simulink model "Quadcopter_Hinfinity"  (R2016b)
settings: Solver=ode45  StartTime=0.0  StopTime=36  RelTol=1e-3  EnableMultiTasking=on
undefined symbols (not defined in the file): A, B, C, D, K1
libraries: simulink x1
settings Model: Creator=Toshiba  LastModifiedBy=AAstudillo
settings DataIOCC: LimitDataPoints=on  SaveFormat=Array  SignalLoggingSaveFormat=ModelDataLogs
settings OptimizationCC: LifeSpan=inf
settings DebuggingCC: SolverPrmCheckMsg=warning  MultiTaskDSMMsg=warning  MultiTaskCondExecSysMsg=none  SFUnexpectedBacktrackingDiag=warning  SFNoUnconditionalDefaultTransitionDiag=warning  SFExecutionAtInitializationDiag=none
settings HardwareCC: ProdBitPerPointer=32  ProdBitPerSizeT=32  ProdBitPerPtrDiffT=32  ProdLargestAtomicFloat=None  ProdIntDivRoundTo=Undefined  ProdEndianess=Unspecified  ProdWordSize=32  ProdHWDeviceType=32-bit Generic
settings ModelReferenceCC: PropagateSignalLabelsOutOfModel=off
settings GRTTargetCC: TargetLangStandard=C89/C90 (ANSI)  GeneratePreprocessorConditionals=Disable all
settings ConfigComp: CovMetricSettings=dw  CovHtmlReporting=on  CovSaveCumulativeToWorkspaceVar=on  CovSaveSingleToWorkspaceVar=on  CovExternalEMLEnable=off

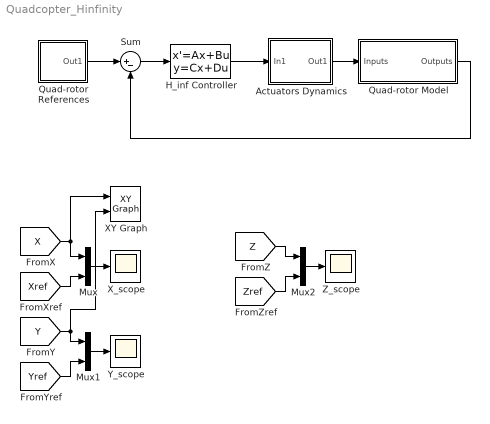
== system Quadcopter_Hinfinity ==
  Actuators Dynamics : Subsystem
  H_inf Controller : StateSpace  A=K1.a  B=K1.b  C=K1.c  D=K1.d  X0=zeros(size(K1.a,1),1)
  Mux : Mux  Inputs=2
  Mux1 : Mux  Inputs=2
  Mux2 : Mux  Inputs=2
  Quad-rotor Model : Subsystem
  Quad-rotor References : Subsystem
  Sum : Sum  Inputs=|+-
  XY Graph : simulink/Sinks/XY Graph  xmin=-1  xmax=1  ymin=-1  ymax=1  st=-1
  X_scope : Scope
  Y_scope : Scope
  Z_scope : Scope
  wires:
  Sum/1 -> H_inf Controller/1
  Quad-rotor References/1(Out1) -> Sum/1
  Quad-rotor Model/1(Outputs) -> Sum/2
  Mux/1 -> X_scope/1
  Mux1/1 -> Y_scope/1
  Mux2/1 -> Z_scope/1
  [X] -> Mux/1, XY Graph/1
  [Xref] -> Mux/2
  [Y] -> Mux1/1, XY Graph/2
  [Yref] -> Mux1/2
  [Z] -> Mux2/1
  [Zref] -> Mux2/2
  H_inf Controller/1 -> Actuators Dynamics/1(In1)
  Actuators Dynamics/1(Out1) -> Quad-rotor Model/1(Inputs)

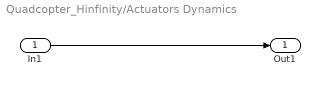
== system Quadcopter_Hinfinity/Actuators Dynamics ==
  In1 : Inport
  Out1 : Outport
  wires:
  In1/1 -> Out1/1

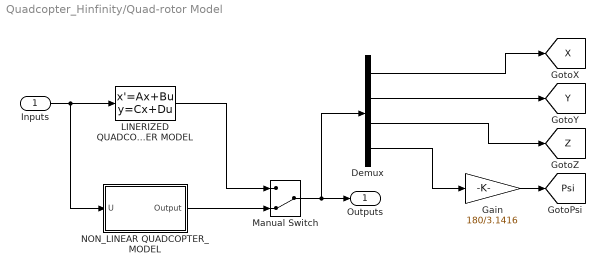
== system Quadcopter_Hinfinity/Quad-rotor Model ==
  Inputs : Inport
  Demux : Demux
  Gain : Gain  Gain=180/3.1416
  LINERIZED QUADCOPTER MODEL : StateSpace  A=A  B=B  C=C  D=D  X0=[0 0 1 0 1.5 0 45*pi/180 0 0 0 0 0]'
  Manual Switch : ManualSwitch  CurrentSetting=0
  NON_LINEAR QUADCOPTER_MODEL : Subsystem
  Outputs : Outport
  tag scope: Psi=global, X=global, Y=global, Z=global
  wires:
  Inputs/1 -> NON_LINEAR QUADCOPTER_MODEL/1(U), LINERIZED QUADCOPTER MODEL/1
  LINERIZED QUADCOPTER MODEL/1 -> Manual Switch/1
  Demux/3 -> [Z]
  Manual Switch/1 -> Outputs/1, Demux/1
  Demux/1 -> [X]
  Demux/2 -> [Y]
  NON_LINEAR QUADCOPTER_MODEL/1("Output ") -> Manual Switch/2
  Gain/1 -> [Psi]
  Demux/4 -> Gain/1

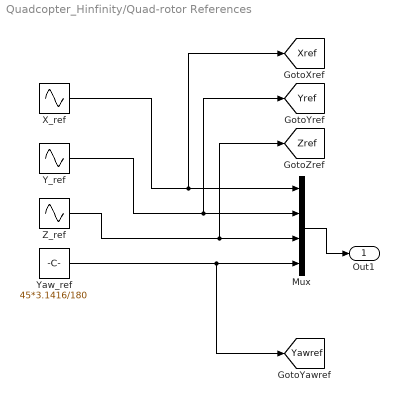
== system Quadcopter_Hinfinity/Quad-rotor References ==
  Mux : Mux
  X_ref : Sin  Frequency=3.141592654*0.1  SampleTime=0
  Y_ref : Sin  Frequency=3.141592654*0.1  Phase=3.141592654/2  SampleTime=0
  Yaw_ref : Constant  Value=45*3.1416/180
  Z_ref : Sin  Bias=1  Frequency=3.141592654*0.05  Phase=3.141592654  SampleTime=0
  Out1 : Outport
  tag scope: Xref=global, Yawref=global, Yref=global, Zref=global
  wires:
  Mux/1 -> Out1/1
  X_ref/1 -> [Xref], Mux/1
  Yaw_ref/1 -> [Yawref], Mux/4
  Z_ref/1 -> [Zref], Mux/3
  Y_ref/1 -> [Yref], Mux/2

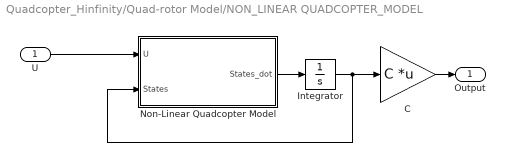
== system Quadcopter_Hinfinity/Quad-rotor Model/NON_LINEAR QUADCOPTER_MODEL ==
  U : Inport
  C : Gain  Gain=C  Multiplication=Matrix(K*u)
  Integrator : Integrator  InitialCondition=[0 0 1 0 1.5 0 45*pi/180 0 0 0 0 0]'
  Non-Linear Quadcopter Model : MATLAB Function  TreatAsAtomicUnit=on
  "Output " : Outport
  wires:
  Non-Linear Quadcopter Model/1(States_dot) -> Integrator/1
  Integrator/1 -> Non-Linear Quadcopter Model/2(States), C/1
  U/1 -> Non-Linear Quadcopter Model/1(U)
  C/1 -> "Output "/1

== matlab function Quadcopter_Hinfinity/Quad-rotor Model/NON_LINEAR QUADCOPTER_MODEL/Non-Linear Quadcopter Model ==
  data: U input; States input; States_dot output
function States_dot  = fcn(U, States)

% Gravity constant
              g = 9.807;

              m = 1.5680;
              Ixx = 0.0135;
              Iyy = 0.0124;
              Izz = 0.0336;

    %Inputs = U, States
    %Outputs = States_dot  
    %States: X dX Y dY Z dZ Psi dPsi Theta dTheta Phi dPhi
    %        1  2 3  4 5  6  7   8     9      10   11  12
    
    U1 = U(1)+m*g;
    U2 = U(2);
    U3 = U(3);
    U4 = U(4);

    dX = States(2);
    ddX = (U1/m)*(cos(States(7))*sin(States(9))*cos(States(11)) + sin(States(7))*sin(States(11)));
    %ddX = -States(10)*States(6) + States(8)*States(4) + g*sin(States(9));
    dY = States(4);
    ddY = (U1/m)*(-sin(States(7))*sin(States(9))*cos(States(11)) + cos(States(7))*sin(States(11)));
    %ddY = States(8)*States(2) - States(12)*States(6) + g*cos(States(9))*sin(States(11));
    dZ = States(6);
    %ddZ = ((U1/m)*cos(States(9))*cos(States(11))) - g;
    ddZ = States(10)*States(2) - States(12)*States(4) - g*cos(States(9))*cos(States(11)) + (U1)/m;
    
    dPsi = States(8);
    ddPsi = (((Ixx-Iyy)/Izz)*States(12)*States(10)) + (U2/Izz);
    dTheta = States(10);
    ddTheta = (((Izz-Ixx)/Iyy)*States(12)*States(8)) + (U3/Iyy);
    dPhi = States(12);
    ddPhi = (((Iyy-Izz)/Ixx)*States(10)*States(8)) + (U4/Ixx);


States_dot = [dX, ddX, dY, ddY, dZ, ddZ, dPsi, ddPsi, dTheta, ddTheta, dPhi, ddPhi]';
